simulink model "LDXIsys"  (R2023a)
settings: Solver=FixedStepDiscrete  StartTime=0.0  StopTime=cin.TimeInfo.End  RelTol=1e-3
values from neighbouring files (symbols this model uses):
  cmax = rows*cols    [LDFItest.m]    (also in LDXItest.m; LXFItest.m; LXFXtest.m; LXXItest.m)
  hmax = ceil((rows*cols/sqrt(12))/pow2(logDPS.stde,8-sbin))    [LDFItest.m]    (also in LDXItest.m; LXFItest.m; LXFXtest.m; LXXItest.m)
  sbin = 4    [LDFItest.m]    (also in LDXItest.m; LXFItest.m; LXFXtest.m; LXXItest.m)
  Ts = 1/(30*rows*cols)    [LDFItest.m]    (also in LDXItest.m; LXFItest.m; LXFXtest.m; LXXItest.m)
libraries: simulink x16, hdlsllib x4
settings Model: Creator=dileepan  LastModifiedBy=dileepan
settings DataIOCC: SaveOutput=off  SignalLogging=off  DSMLogging=off  SaveTime=off  ReturnWorkspaceOutputs=off

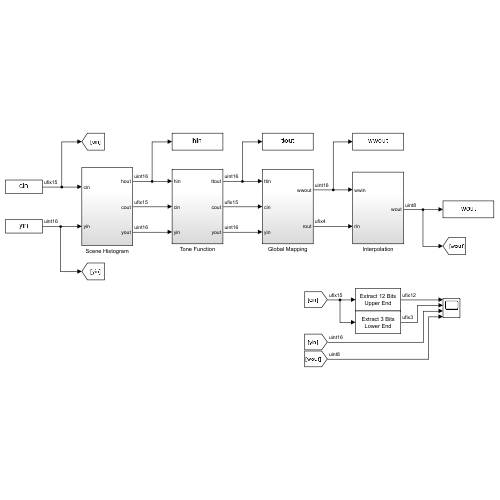
[thumbnail: Simulink's stored preview of the top-level diagram]
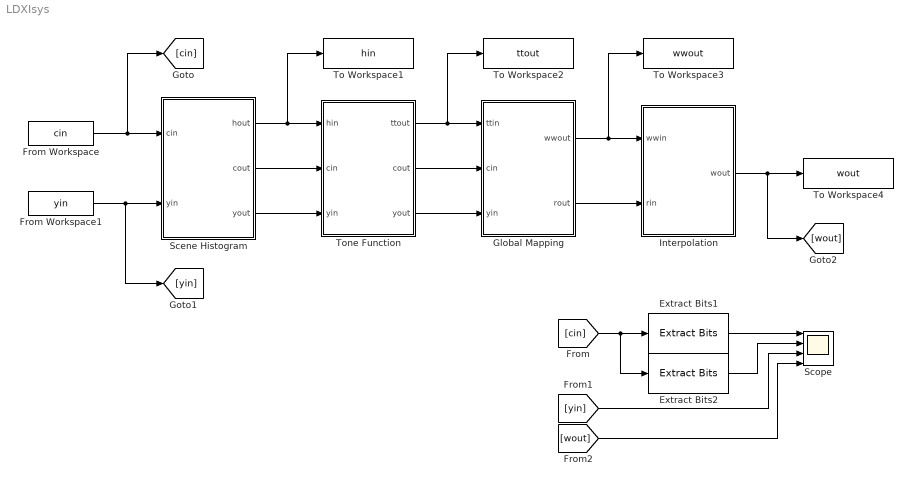
== system LDXIsys ==
  Extract Bits1 : simulink/Logic and Bit Operations/Extract Bits  bitsToExtract=Range starting with most significant bit  numBits=16-sbin  bitIdxRange=2+[0 15-sbin]  outScalingMode=Treat bit field as an integer
  Extract Bits2 : simulink/Logic and Bit Operations/Extract Bits  bitsToExtract=Range ending with least significant bit  numBits=3  bitIdxRange=[0 1]  outScalingMode=Treat bit field as an integer
  From Workspace : FromWorkspace  VariableName=cin  SampleTime=Ts  Interpolate=off  OutputAfterFinalValue=Setting to zero
  From Workspace1 : FromWorkspace  VariableName=yin  SampleTime=Ts  Interpolate=off  OutputAfterFinalValue=Setting to zero
  Global Mapping : Subsystem
  Interpolation : Subsystem
  Scene Histogram : Subsystem
  Scope : Scope  NumInputPorts=4
  To Workspace1 : ToWorkspace  VariableName=hin  SaveFormat=Timeseries  SampleTime=-1
      settings: Save2DSignal=2-D array (concatenate along first dimension)
  To Workspace2 : ToWorkspace  VariableName=ttout  SaveFormat=Timeseries  SampleTime=-1
      settings: Save2DSignal=2-D array (concatenate along first dimension)
  To Workspace3 : ToWorkspace  VariableName=wwout  SaveFormat=Timeseries  SampleTime=-1
      settings: Save2DSignal=2-D array (concatenate along first dimension)
  To Workspace4 : ToWorkspace  VariableName=wout  SaveFormat=Timeseries  SampleTime=-1
      settings: Save2DSignal=2-D array (concatenate along first dimension)
  Tone Function : Subsystem
  wires:
  From Workspace/1 -> Scene Histogram/1(cin), [cin]
  From Workspace1/1 -> Scene Histogram/2(yin), [yin]
  [cin] -> Extract Bits2/1, Extract Bits1/1
  Extract Bits1/1 -> Scope/1
  Extract Bits2/1 -> Scope/2
  [yin] -> Scope/3
  [wout] -> Scope/4
  Scene Histogram/1(hout) -> Tone Function/1(hin), To Workspace1/1
  Global Mapping/1(wwout) -> Interpolation/1(wwin), To Workspace3/1
  Global Mapping/2(rout) -> Interpolation/2(rin)
  Interpolation/1(wout) -> [wout], To Workspace4/1
  Scene Histogram/3(yout) -> Tone Function/3(yin)
  Scene Histogram/2(cout) -> Tone Function/2(cin)
  Tone Function/3(yout) -> Global Mapping/3(yin)
  Tone Function/2(cout) -> Global Mapping/2(cin)
  Tone Function/1(ttout) -> To Workspace2/1, Global Mapping/1(ttin)

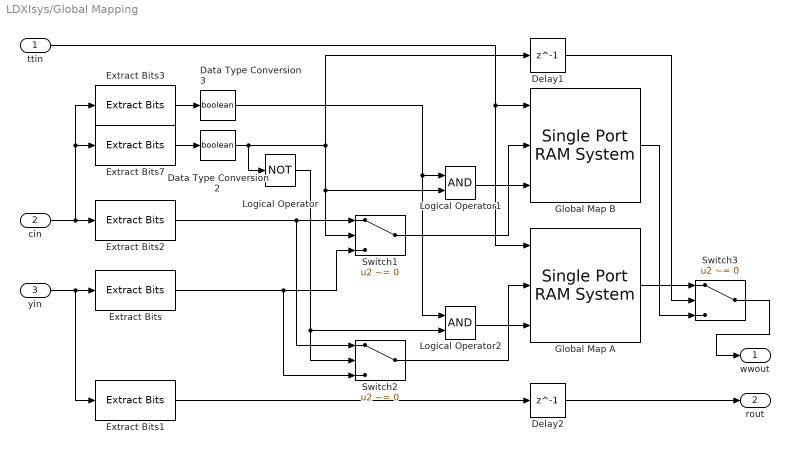
== system LDXIsys/Global Mapping ==
  ttin : Inport
  cin : Inport  Port=2
  yin : Inport  Port=3
  Data Type Conversion2 : DataTypeConversion  OutDataTypeStr=boolean  ConvertRealWorld=Stored Integer (SI)  SaturateOnIntegerOverflow=off  RndMeth=Floor
  Data Type Conversion3 : DataTypeConversion  OutDataTypeStr=boolean  ConvertRealWorld=Stored Integer (SI)  SaturateOnIntegerOverflow=off  RndMeth=Floor
  Delay1 : Delay  DelayLength=1
  Delay2 : Delay  DelayLength=1
  Extract Bits : simulink/Logic and Bit Operations/Extract Bits  bitsToExtract=Range starting with most significant bit  numBits=16-sbin  bitIdxRange=[0 7]  outScalingMode=Treat bit field as an integer
  Extract Bits1 : simulink/Logic and Bit Operations/Extract Bits  bitsToExtract=Range ending with least significant bit  numBits=sbin  bitIdxRange=0  outScalingMode=Treat bit field as an integer
  Extract Bits2 : simulink/Logic and Bit Operations/Extract Bits  bitsToExtract=Range starting with most significant bit  numBits=16-sbin  bitIdxRange=[2 17-sbin]  outScalingMode=Treat bit field as an integer
  Extract Bits3 : simulink/Logic and Bit Operations/Extract Bits  bitsToExtract=Range of bits  numBits=2  bitIdxRange=1  outScalingMode=Treat bit field as an integer
  Extract Bits7 : simulink/Logic and Bit Operations/Extract Bits  bitsToExtract=Range of bits  numBits=1  bitIdxRange=0  outScalingMode=Treat bit field as an integer
  Global Map A : hdlsllib/HDL RAMs/Single Port RAM System  RAMType=Single port  WriteOutputValue=New data  RAMInitialValue=0  SimulateUsing=Code generation
  Global Map B : hdlsllib/HDL RAMs/Single Port RAM System  RAMType=Single port  WriteOutputValue=New data  RAMInitialValue=0  SimulateUsing=Code generation
  Logical Operator : Logic  Operator=NOT  IconShape=distinctive  AllPortsSameDT=off  OutDataTypeStr=boolean
  Logical Operator1 : Logic  AllPortsSameDT=off  OutDataTypeStr=boolean
  Logical Operator2 : Logic  AllPortsSameDT=off  OutDataTypeStr=boolean
  Switch1 : Switch  Criteria=u2 ~= 0  SaturateOnIntegerOverflow=off  InputSameDT=off
  Switch2 : Switch  Criteria=u2 ~= 0  SaturateOnIntegerOverflow=off  InputSameDT=off
  Switch3 : Switch  Criteria=u2 ~= 0  SaturateOnIntegerOverflow=off  InputSameDT=off
  wwout : Outport
  rout : Outport  Port=2
  wires:
  Delay2/1 -> rout/1
  Delay1/1 -> Switch3/2
  Global Map B/1 -> Switch3/3
  Switch3/1 -> wwout/1
  ttin/1 -> Global Map B/1, Global Map A/1
  cin/1 -> Extract Bits2/1, Extract Bits3/1, Extract Bits7/1
  Extract Bits1/1 -> Delay2/1
  Extract Bits/1 -> Switch2/3, Switch1/3
  Data Type Conversion3/1 -> Logical Operator1/1, Logical Operator2/1
  Extract Bits2/1 -> Switch2/1, Switch1/1
  Switch1/1 -> Global Map B/2
  Logical Operator1/1 -> Global Map B/3
  Data Type Conversion2/1 -> Logical Operator/1, Delay1/1, Switch1/2, Logical Operator1/2
  Switch2/1 -> Global Map A/2
  Logical Operator/1 -> Logical Operator2/2, Switch2/2
  Extract Bits7/1 -> Data Type Conversion2/1
  yin/1 -> Extract Bits1/1, Extract Bits/1
  Extract Bits3/1 -> Data Type Conversion3/1
  Global Map A/1 -> Switch3/1
  Logical Operator2/1 -> Global Map A/3

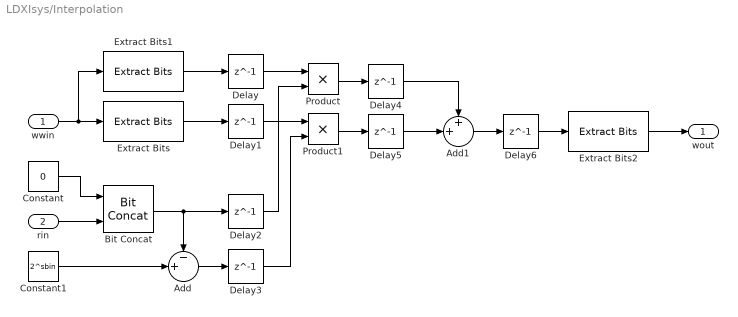
== system LDXIsys/Interpolation ==
  wwin : Inport
  rin : Inport  Port=2
  Add : Sum  Inputs=-+|  OutDataTypeStr=Inherit: Same as accumulator
  Add1 : Sum  Inputs=++|  OutDataTypeStr=Inherit: Same as accumulator
  Bit Concat : hdlsllib/Logic and Bit Operations/Bit Concat  numInputs=2
  Constant : Constant  Value=0  OutDataTypeStr=fixdt(0,1,0)  SampleTime=Ts
  Constant1 : Constant  Value=2^sbin  OutDataTypeStr=fixdt(0,sbin+1,0)  SampleTime=Ts
  Delay{,1..6} (7 alike) : Delay  DelayLength=1
  Extract Bits : simulink/Logic and Bit Operations/Extract Bits  bitsToExtract=Lower half  numBits=8  bitIdxRange=[0 7]  outScalingMode=Treat bit field as an integer
  Extract Bits1 : simulink/Logic and Bit Operations/Extract Bits  bitsToExtract=Upper half  numBits=8  bitIdxRange=[0 7]  outScalingMode=Treat bit field as an integer
  Extract Bits2 : simulink/Logic and Bit Operations/Extract Bits  bitsToExtract=Range of bits  numBits=8  bitIdxRange=[0 7]+sbin  outScalingMode=Treat bit field as an integer
  Product : Product  OutDataTypeStr=fixdt(0,8+sbin+1,0)
  Product1 : Product  OutDataTypeStr=fixdt(0,8+sbin+1,0)
  wout : Outport
  wires:
  Constant1/1 -> Add/2
  Product/1 -> Delay4/1
  Extract Bits1/1 -> Delay/1
  Delay6/1 -> Extract Bits2/1
  rin/1 -> Bit Concat/2
  Add1/1 -> Delay6/1
  Delay5/1 -> Add1/2
  Delay/1 -> Product/1
  Extract Bits/1 -> Delay1/1
  Product1/1 -> Delay5/1
  Delay1/1 -> Product1/1
  Delay4/1 -> Add1/1
  Add/1 -> Delay3/1
  Delay3/1 -> Product1/2
  Delay2/1 -> Product/2
  Extract Bits2/1 -> wout/1
  wwin/1 -> Extract Bits1/1, Extract Bits/1
  Constant/1 -> Bit Concat/1
  Bit Concat/1 -> Delay2/1, Add/1

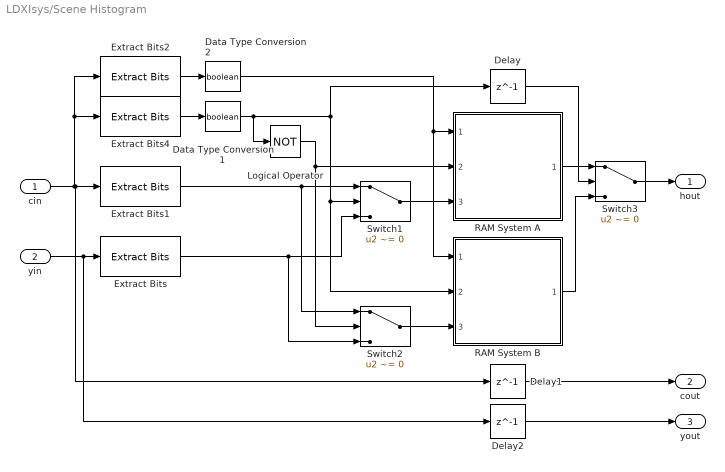
== system LDXIsys/Scene Histogram ==
  cin : Inport
  yin : Inport  Port=2
  Data Type Conversion1 : DataTypeConversion  OutDataTypeStr=boolean  ConvertRealWorld=Stored Integer (SI)  SaturateOnIntegerOverflow=off  RndMeth=Floor
  Data Type Conversion2 : DataTypeConversion  OutDataTypeStr=boolean  ConvertRealWorld=Stored Integer (SI)  SaturateOnIntegerOverflow=off  RndMeth=Floor
  Delay : Delay  DelayLength=1
  Delay1 : Delay  DelayLength=1
  Delay2 : Delay  DelayLength=1
  Extract Bits : simulink/Logic and Bit Operations/Extract Bits  bitsToExtract=Range starting with most significant bit  numBits=16-sbin  bitIdxRange=[0 7]  outScalingMode=Treat bit field as an integer
  Extract Bits1 : simulink/Logic and Bit Operations/Extract Bits  bitsToExtract=Range starting with most significant bit  numBits=16-sbin  bitIdxRange=[2 17-sbin]  outScalingMode=Treat bit field as an integer
  Extract Bits2 : simulink/Logic and Bit Operations/Extract Bits  bitsToExtract=Range of bits  numBits=2  bitIdxRange=1  outScalingMode=Treat bit field as an integer
  Extract Bits4 : simulink/Logic and Bit Operations/Extract Bits  bitsToExtract=Range of bits  numBits=1  bitIdxRange=0  outScalingMode=Treat bit field as an integer
  Logical Operator : Logic  Operator=NOT  IconShape=distinctive  AllPortsSameDT=off  OutDataTypeStr=boolean
  RAM System A : Subsystem  ReferencedSubsystem=RAMsys
  RAM System B : Subsystem  ReferencedSubsystem=RAMsys
  Switch1 : Switch  Criteria=u2 ~= 0  SaturateOnIntegerOverflow=off  InputSameDT=off
  Switch2 : Switch  Criteria=u2 ~= 0  SaturateOnIntegerOverflow=off  InputSameDT=off
  Switch3 : Switch  Criteria=u2 ~= 0  SaturateOnIntegerOverflow=off  InputSameDT=off
  hout : Outport
  cout : Outport  Port=2
  yout : Outport  Port=3
  wires:
  Extract Bits2/1 -> Data Type Conversion2/1
  RAM System A/1 -> Switch3/1
  Switch1/1 -> RAM System A/3
  Extract Bits1/1 -> Switch2/1, Switch1/1
  Extract Bits4/1 -> Data Type Conversion1/1
  cin/1 -> Delay1/1, Extract Bits1/1, Extract Bits4/1, Extract Bits2/1
  Switch3/1 -> hout/1
  Logical Operator/1 -> Switch2/2, RAM System A/2
  Extract Bits/1 -> Switch2/3, Switch1/3
  Data Type Conversion2/1 -> RAM System B/1, RAM System A/1
  yin/1 -> Delay2/1, Extract Bits/1
  Delay2/1 -> yout/1
  Data Type Conversion1/1 -> Logical Operator/1, Delay/1, RAM System B/2, Switch1/2
  Delay/1 -> Switch3/2
  RAM System B/1 -> Switch3/3
  Switch2/1 -> RAM System B/3
  Delay1/1 -> cout/1

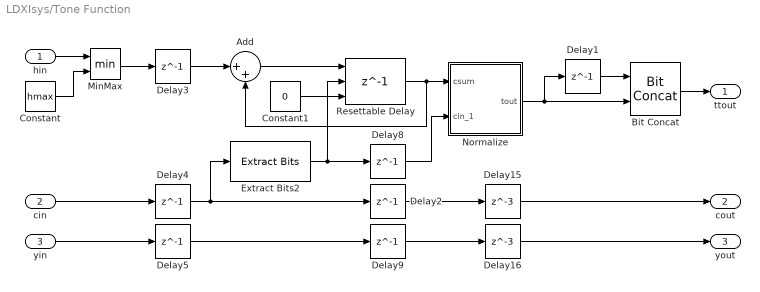
== system LDXIsys/Tone Function ==
  hin : Inport
  cin : Inport  Port=2
  yin : Inport  Port=3
  Add : Sum  Inputs=|++  OutDataTypeStr=Inherit: Same as accumulator
  Bit Concat : hdlsllib/Logic and Bit Operations/Bit Concat  numInputs=2
  Constant : Constant  Value=hmax  OutDataTypeStr=fixdt(0,ceil(log2(rows*cols)),0)  SampleTime=Ts
  Constant1 : Constant  Value=0  OutDataTypeStr=fixdt(0,bitc,0)  SampleTime=Ts
  Delay{1..5,8..9} (7 alike) : Delay  DelayLength=1
  Delay15 : Delay  DelayLength=3
  Delay16 : Delay  DelayLength=3
  Extract Bits2 : simulink/Logic and Bit Operations/Extract Bits  bitsToExtract=Range of bits  numBits=2  bitIdxRange=1  outScalingMode=Treat bit field as an integer
  MinMax : MinMax  Inputs=2
  Normalize : Subsystem
  Resettable Delay : Delay  DelayLength=1  InitialConditionSource=Input port  ExternalReset=Rising
      settings: InputPortMap=u0,r5,p4
  ttout : Outport
  cout : Outport  Port=2
  yout : Outport  Port=3
  wires:
  Delay1/1 -> Bit Concat/1
  hin/1 -> MinMax/1
  Delay2/1 -> Delay15/1
  Delay5/1 -> Delay9/1
  Add/1 -> Resettable Delay/1
  cin/1 -> Delay4/1
  Resettable Delay/1 -> Normalize/1(csum), Add/2
  Delay15/1 -> cout/1
  Delay3/1 -> Add/1
  Normalize/1(tout) -> Bit Concat/2, Delay1/1
  MinMax/1 -> Delay3/1
  Delay4/1 -> Delay2/1, Extract Bits2/1
  Extract Bits2/1 -> Resettable Delay/2, Delay8/1
  Delay16/1 -> yout/1
  yin/1 -> Delay5/1
  Constant/1 -> MinMax/2
  Delay9/1 -> Delay16/1
  Constant1/1 -> Resettable Delay/3
  Bit Concat/1 -> ttout/1
  Delay8/1 -> Normalize/2(cin_1)

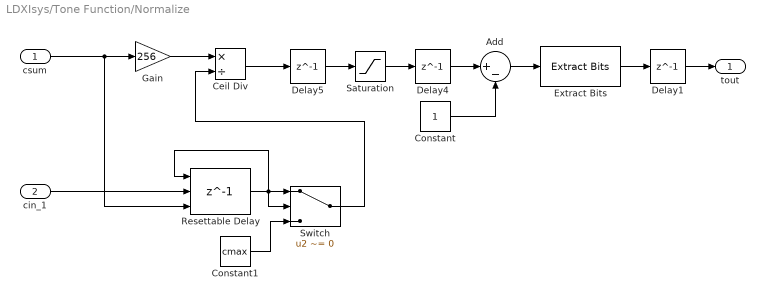
== system LDXIsys/Tone Function/Normalize ==
  csum : Inport
  cin_1 : Inport  Port=2
  Add : Sum  Inputs=|+-  OutDataTypeStr=Inherit: Same as accumulator
  Ceil Div : Product  Inputs=*/  OutDataTypeStr=fixdt(0,9,0)  RndMeth=Ceiling
  Constant : Constant  OutDataTypeStr=fixdt(0,1,0)  SampleTime=Ts
  Constant1 : Constant  Value=cmax  OutDataTypeStr=fixdt(0,bitc,0)  SampleTime=Ts
  Delay1 : Delay  DelayLength=1
  Delay4 : Delay  DelayLength=1
  Delay5 : Delay  DelayLength=1
  Extract Bits : simulink/Logic and Bit Operations/Extract Bits  bitsToExtract=Range ending with least significant bit  numBits=8  bitIdxRange=[0 7]  outScalingMode=Treat bit field as an integer
      settings: LibrarySourceBlock=|
      | hdlsllib/Logic and Bit
      | Operations/Extract Bits
  Gain : Gain  Gain=256  OutDataTypeStr=fixdt(0,bitc+8,0)
  Resettable Delay : Delay  DelayLength=1  InitialConditionSource=Input port  ExternalReset=Falling
      settings: InputPortMap=u0,r5,p4
  Saturation : Saturate  UpperLimit=256  LowerLimit=1
  Switch : Switch  Criteria=u2 ~= 0  SaturateOnIntegerOverflow=off  InputSameDT=off
  tout : Outport
  wires:
  csum/1 -> Resettable Delay/3, Gain/1
  Resettable Delay/1 -> Switch/1, Switch/2, Resettable Delay/1
  cin_1/1 -> Resettable Delay/2
  Delay1/1 -> tout/1
  Constant/1 -> Add/2
  Delay4/1 -> Add/1
  Gain/1 -> Ceil Div/1
  Add/1 -> Extract Bits/1
  Extract Bits/1 -> Delay1/1
  Ceil Div/1 -> Delay5/1
  Delay5/1 -> Saturation/1
  Saturation/1 -> Delay4/1
  Constant1/1 -> Switch/3
  Switch/1 -> Ceil Div/2
